simulink model "KUKAKR70"  (R2022b)
settings: Solver=ode4  StartTime=0.0  StopTime=TrajTime  FixedStep=Ts  RelTol=1e-3
values from neighbouring files (symbols this model uses):
  C = reshape([mt1,mt2,mt3,mt4,mt5,mt6,mt7,mt8,mt9,mt10,mt11,mt12,mt13,mt14,mt15,mt16,mt17],6,6)    [KR70CMatrix.m]
  X = 1200    [KR70ComputedTorque.m]
  Y = 1200    [KR70ComputedTorque.m]
  Z = 1200    [KR70ComputedTorque.m]
libraries: sm_lib x24, nesl_utility x19, simulink_extras x3
settings Model: Creator=Aboudi  LastModifiedBy=revdu
settings SolverCC: AlgebraicLoopSolver=TrustRegion
settings OptimizationCC: EnhancedBackFolding=on  PassReuseOutputArgsAs=Individual arguments  ZeroExternalMemoryAtStartup=off  ZeroInternalMemoryAtStartup=off  MaxStackSize=64  OptimizeBlockOrder=speed  DifferentSizesBufferReuse=on  OptimizationCustomize=off  EfficientTunableParamExpr=on
settings DebuggingCC: ParameterTunabilityLossMsg=error  UnconnectedInputMsg=warning  UnconnectedOutputMsg=warning  UnconnectedLineMsg=warning  SFMachineParentedDataDiag=warning
settings HardwareCC: ProdBitPerPointer=32  ProdBitPerSizeT=32  ProdBitPerPtrDiffT=32  ProdLargestAtomicFloat=None  ProdIntDivRoundTo=Undefined  ProdEndianess=Unspecified  ProdWordSize=32  ProdHWDeviceType=Generic->Unspecified (assume 32-bit Generic)
settings ModelReferenceCC: EnableRefExpFcnMdlSchedulingChecks=on
settings SFSimCC: MATLABDynamicMemAlloc=off
settings RTWCC: Description=Embedded Coder  SystemTargetFile=ert.tlc  HardwareBoard=Robot Operating System (ROS)  TLCOptions="-aInlineSetEventsForThisBaseRateFcn=TLC_FALSE -aSuppressMultiTaskScheduler=TLC_FALSE  -aRateBasedStepFcn=0"  TemplateMakefile=ert_default_tmf  Toolchain=Catkin  TargetLang=C++
settings CodeAppCC: ForceParamTrailComments=on  IgnoreCustomStorageClasses=off  OperatorAnnotations=on  SimulinkDataObjDesc=on  SFDataObjDesc=on  InsertBlockDesc=on
settings ExplorerConfigSet: InternalSimMechanicsExplorerSettings="<ExplorerConfiguration><canonicalview>aerospace</canonicalview><AnimationSetting><BasePlaybackSpeed>1.0</BasePlaybackSpeed><PlaybackSpeedFactor>1.0</PlaybackSpeedFactor></AnimationSetting><TilePanel><TileInfo><Tiles Columns=\"1\" Count=\"1\" Rows=\"1\"><Column Weight=\"1\"/><Row Weight=\"1\"/><Tile Height=\"1\" Width=\"1\" X=\"0\" Y=\"0\"/></Tiles></TileInfo><SceneInfo><SceneViewer><BGColor><R>0.60000002384185791</R><G>0.60000002384185791</G><B>0.60000002384185791</B></BGColor><Camera><DoPerspective>off</DoPerspective><Position><X>3.02357332435470916</X><Y>-3.32920549020346535</Y><Z>2.30639573599890824</Z></Position><Center><X>-0.276547744173664067</X><Y>0.35019971331948252</Y><Z>-0.00815298373152223421</Z></Center><Up><X>-0.335011191369486205</X><Y>0.267785677359949403</Y><Z>0.903359470342825488</Z></Up><ViewLimDist>1</ViewLimDist><YLim>2.19360700639605977</YLim><XLim>3.27073690415556007</XLim></Camera></SceneViewer></SceneInfo></TilePanel><MechEditorPanel><Cameras/><GfxPanelCameraMap/><VideoCreator><PlaybackSpeedRatio>1.0</PlaybackSpeedRatio><FrameRate>30</FrameRate><VideoFormat>Motion JPEG AVI</VideoFormat><FrameSize>auto</FrameSize></VideoCreator></MechEditorPanel></ExplorerConfiguration>"

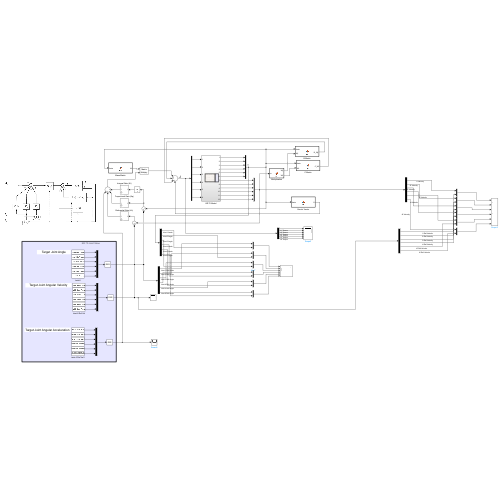
[thumbnail: Simulink's stored preview of the top-level diagram]
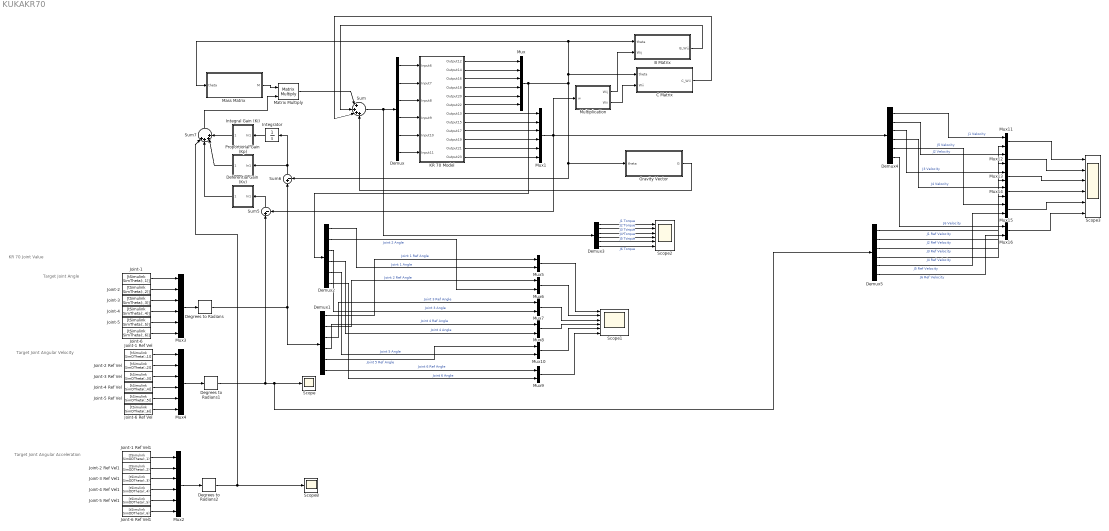
== system KUKAKR70 ==
  note: KR 70 Joint Value
  note: Target Joint Angular Velocity
  note: Target Joint Angle
  note: Target Joint Angular Acceleration
  B Matrix : MATLAB Function  TreatAsAtomicUnit=on
  C Matrix : MATLAB Function  TreatAsAtomicUnit=on
  Deferential Gain (Kv) : Subsystem  mask{Kv1=1e2, Kv2=1e2, Kv3=1e2, Kv4=1e2, Kv5=1e2, Kv6=1e3}
  Degrees to Radians : simulink_extras/Transformations/Degrees to Radians
  Degrees to Radians1 : simulink_extras/Transformations/Degrees to Radians
  Degrees to Radians2 : simulink_extras/Transformations/Degrees to Radians
  Demux{,1..5} (6 alike) : Demux  Outputs=6
  Gravity Vector : MATLAB Function  TreatAsAtomicUnit=on
  Integral Gain (Ki) : Subsystem  mask{Ki1=2e3, Ki2=2e3, Ki3=1e3, Ki4=1e2, Ki5=1e2, Ki6=1e3}
  Integrator : Integrator
  Joint-1 : FromWorkspace  VariableName=[tSimulink SimTheta(:,1)]  SampleTime=-1  OutputAfterFinalValue=Holding final value
  Joint-1 Ref Vel : FromWorkspace  VariableName=[tSimulink SimDTheta(:,1)]  SampleTime=-1  OutputAfterFinalValue=Holding final value
  Joint-1 Ref Vel1 : FromWorkspace  VariableName=[tSimulink SimDDTheta(:,1)]  SampleTime=-1  OutputAfterFinalValue=Holding final value
  Joint-2 : FromWorkspace  VariableName=[tSimulink SimTheta(:,2)]  SampleTime=-1  OutputAfterFinalValue=Holding final value
  Joint-2 Ref Vel : FromWorkspace  VariableName=[tSimulink SimDTheta(:,2)]  SampleTime=-1  OutputAfterFinalValue=Holding final value
  Joint-2 Ref Vel1 : FromWorkspace  VariableName=[tSimulink SimDDTheta(:,2)]  SampleTime=-1  OutputAfterFinalValue=Holding final value
  Joint-3 : FromWorkspace  VariableName=[tSimulink SimTheta(:,3)]  SampleTime=-1  OutputAfterFinalValue=Holding final value
  Joint-3 Ref Vel : FromWorkspace  VariableName=[tSimulink SimDTheta(:,3)]  SampleTime=-1  OutputAfterFinalValue=Holding final value
  Joint-3 Ref Vel1 : FromWorkspace  VariableName=[tSimulink SimDDTheta(:,3)]  SampleTime=-1  OutputAfterFinalValue=Holding final value
  Joint-4 : FromWorkspace  VariableName=[tSimulink SimTheta(:,4)]  SampleTime=-1  OutputAfterFinalValue=Holding final value
  Joint-4 Ref Vel : FromWorkspace  VariableName=[tSimulink SimDTheta(:,4)]  SampleTime=-1  OutputAfterFinalValue=Holding final value
  Joint-4 Ref Vel1 : FromWorkspace  VariableName=[tSimulink SimDDTheta(:,4)]  SampleTime=-1  OutputAfterFinalValue=Holding final value
  Joint-5 : FromWorkspace  VariableName=[tSimulink SimTheta(:,5)]  SampleTime=-1  OutputAfterFinalValue=Holding final value
  Joint-5 Ref Vel : FromWorkspace  VariableName=[tSimulink SimDTheta(:,5)]  SampleTime=-1  OutputAfterFinalValue=Holding final value
  Joint-5 Ref Vel1 : FromWorkspace  VariableName=[tSimulink SimDDTheta(:,5)]  SampleTime=-1  OutputAfterFinalValue=Holding final value
  Joint-6 : FromWorkspace  VariableName=[tSimulink SimTheta(:,6)]  SampleTime=-1  OutputAfterFinalValue=Holding final value
  Joint-6 Ref Vel : FromWorkspace  VariableName=[tSimulink SimDTheta(:,6)]  SampleTime=-1  OutputAfterFinalValue=Holding final value
  Joint-6 Ref Vel1 : FromWorkspace  VariableName=[tSimulink SimDDTheta(:,6)]  SampleTime=-1  OutputAfterFinalValue=Holding final value
  KR 70 Model : Subsystem
  Mass Matrix : MATLAB Function  TreatAsAtomicUnit=on
  Matrix Multiply : Product  Multiplication=Matrix(*)
  Multiplication : MATLAB Function  TreatAsAtomicUnit=on
  Mux{,1..4} (5 alike) : Mux  Inputs=6
  Mux{5..16} (12 alike) : Mux  Inputs=2
  Proportional Gain (Kp) : Subsystem  mask{K1=1e3, K2=1e3, K3=1e3, K4=3e3, K5=1e3, K6=1e6}
  Scope : Scope
  Scope1 : Scope  NumInputPorts=6
  Scope2 : Scope  NumInputPorts=6
  Scope3 : Scope  NumInputPorts=6
  Scope8 : Scope
  Sum : Sum  Inputs=|++++
  Sum5 : Sum  Inputs=|+-
  Sum6 : Sum  Inputs=|+-
  Sum7 : Sum  Inputs=|++++
  wires:
  KR 70 Model/1(Output12) -> Mux/1
  KR 70 Model/7(Output13) -> Mux1/1
  KR 70 Model/8(Output15) -> Mux1/2
  KR 70 Model/9(Output17) -> Mux1/3
  KR 70 Model/10(Output19) -> Mux1/4
  KR 70 Model/11(Output21) -> Mux1/5
  KR 70 Model/12(Output23) -> Mux1/6
  Mux1/1 -> Sum5/2, Demux4/1, Multiplication/1(w)
  Mux/1 -> Demux2/1, C Matrix/1(theta), Mass Matrix/1(theta), B Matrix/1(theta), Sum6/2, Gravity Vector/1(theta)
  Mass Matrix/1(M) -> Matrix Multiply/1
  Demux/1 -> KR 70 Model/1(Input6)
  Demux/2 -> KR 70 Model/2(Input7)
  Demux/3 -> KR 70 Model/3(Input8)
  Demux/4 -> KR 70 Model/4(Input9)
  Demux/5 -> KR 70 Model/5(Input10)
  Demux/6 -> KR 70 Model/6(Input11)
  Matrix Multiply/1 -> Sum/1
  Sum/1 -> Demux3/1, Demux/1
  Multiplication/2(Wii) -> C Matrix/2(Wii)
  Multiplication/1(Wij) -> B Matrix/2(Wij)
  Gravity Vector/1(G) -> Sum/4
  Sum6/1 -> Proportional Gain (Kp)/1(In1), Integrator/1
  Sum5/1 -> Deferential Gain (Kv)/1(In1)
  Integrator/1 -> Integral Gain (Ki)/1(In1)
  Sum7/1 -> Matrix Multiply/2
  C Matrix/1(C_Wii) -> Sum/3
  B Matrix/1(B_Wij) -> Sum/2
  Mux3/1 -> Degrees to Radians/1
  Deferential Gain (Kv)/1(Out1) -> Sum7/2
  Degrees to Radians2/1 -> Scope8/1, Sum7/1
  Mux4/1 -> Degrees to Radians1/1
  Integral Gain (Ki)/1(Out1) -> Sum7/4
  Proportional Gain (Kp)/1(Out1) -> Sum7/3
  Joint-1/1 -> Mux3/1
  Joint-2/1 -> Mux3/2
  Joint-3/1 -> Mux3/3
  Joint-4/1 -> Mux3/4
  Joint-5/1 -> Mux3/5
  Joint-6/1 -> Mux3/6
  KR 70 Model/2(Output14) -> Mux/2
  KR 70 Model/3(Output16) -> Mux/3
  KR 70 Model/4(Output18) -> Mux/4
  KR 70 Model/5(Output20) -> Mux/5
  KR 70 Model/6(Output22) -> Mux/6
  Joint-4 Ref Vel/1 -> Mux4/4
  Joint-5 Ref Vel/1 -> Mux4/5
  Joint-1 Ref Vel/1 -> Mux4/1
  Joint-6 Ref Vel/1 -> Mux4/6
  Joint-2 Ref Vel/1 -> Mux4/2
  Joint-3 Ref Vel/1 -> Mux4/3
  Degrees to Radians/1 -> Sum6/1, Demux1/1
  Degrees to Radians1/1 -> Sum5/1, Demux5/1, Scope/1
  Mux2/1 -> Degrees to Radians2/1
  Joint-2 Ref Vel1/1 -> Mux2/2
  Joint-3 Ref Vel1/1 -> Mux2/3
  Joint-6 Ref Vel1/1 -> Mux2/6
  Joint-4 Ref Vel1/1 -> Mux2/4
  Joint-1 Ref Vel1/1 -> Mux2/1
  Joint-5 Ref Vel1/1 -> Mux2/5
  Demux1/1 -> Mux5/1  "Joint 1 Ref Angle"
  Demux2/1 -> Mux5/2  "Joint 1 Angle"
  Mux5/1 -> Scope1/1
  Mux6/1 -> Scope1/2
  Mux7/1 -> Scope1/3
  Mux8/1 -> Scope1/4
  Mux10/1 -> Scope1/5
  Mux9/1 -> Scope1/6
  Demux1/2 -> Mux6/1  "Joint 2 Ref Angle"
  Demux1/3 -> Mux7/1  "Joint 3 Ref Angle"
  Demux1/4 -> Mux8/1  "Joint 4 Ref Angle"
  Demux1/5 -> Mux10/1  "Joint 5 Ref Angle"
  Demux1/6 -> Mux9/1  "Joint 6 Ref Angle"
  Demux2/2 -> Mux6/2  "Joint 2 Angle"
  Demux2/3 -> Mux7/2  "Joint 3 Angle"
  Demux2/4 -> Mux8/2  "Joint 4 Angle"
  Demux2/5 -> Mux10/2  "Joint 5 Angle"
  Demux2/6 -> Mux9/2  "Joint 6 Angle"
  Demux3/1 -> Scope2/1  "J1 Torque"
  Demux3/2 -> Scope2/2  "J2 Torque"
  Demux3/3 -> Scope2/3  "J3 Torque"
  Demux3/4 -> Scope2/4  "J4 Torque"
  Demux3/5 -> Scope2/5  "J5 Torque"
  Demux3/6 -> Scope2/6  "J6 Torque"
  Mux11/1 -> Scope3/1
  Mux12/1 -> Scope3/2
  Mux13/1 -> Scope3/3
  Mux14/1 -> Scope3/4
  Mux15/1 -> Scope3/5
  Mux16/1 -> Scope3/6
  Demux4/1 -> Mux11/1  "J1 Velocity"
  Demux4/2 -> Mux12/1  "J2 Velocity"
  Demux4/3 -> Mux13/1  "J3 Velocity"
  Demux4/4 -> Mux14/1  "J4 Velocity"
  Demux4/5 -> Mux15/1  "J5 Velocity"
  Demux4/6 -> Mux16/1  "J6 Velocity"
  Demux5/1 -> Mux11/2  "J1 Ref Velocity"
  Demux5/2 -> Mux12/2  "J2 Ref Velocity"
  Demux5/3 -> Mux13/2  "J3 Ref Velocity"
  Demux5/4 -> Mux14/2  "J4 Ref Velocity"
  Demux5/5 -> Mux15/2  "J5 Ref Velocity"
  Demux5/6 -> Mux16/2  "J6 Ref Velocity"

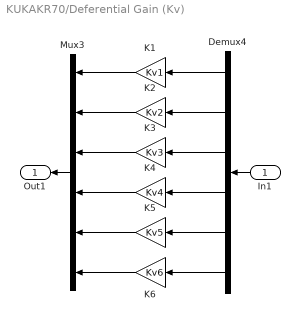
== system KUKAKR70/Deferential Gain (Kv) ==
  In1 : Inport
  Demux4 : Demux  Outputs=6
  K1 : Gain  Gain=Kv1
  K2 : Gain  Gain=Kv2
  K3 : Gain  Gain=Kv3
  K4 : Gain  Gain=Kv4
  K5 : Gain  Gain=Kv5
  K6 : Gain  Gain=Kv6
  Mux3 : Mux  Inputs=6
  Out1 : Outport
  wires:
  Demux4/3 -> K3/1
  K2/1 -> Mux3/2
  K1/1 -> Mux3/1
  K6/1 -> Mux3/6
  Demux4/2 -> K2/1
  Demux4/5 -> K5/1
  Demux4/4 -> K4/1
  Demux4/1 -> K1/1
  K4/1 -> Mux3/4
  Demux4/6 -> K6/1
  K3/1 -> Mux3/3
  K5/1 -> Mux3/5
  In1/1 -> Demux4/1
  Mux3/1 -> Out1/1

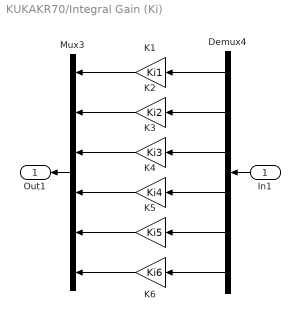
== system KUKAKR70/Integral Gain (Ki) ==
  In1 : Inport
  Demux4 : Demux  Outputs=6
  K1 : Gain  Gain=Ki1
  K2 : Gain  Gain=Ki2
  K3 : Gain  Gain=Ki3
  K4 : Gain  Gain=Ki4
  K5 : Gain  Gain=Ki5
  K6 : Gain  Gain=Ki6
  Mux3 : Mux  Inputs=6
  Out1 : Outport
  wires:
  Demux4/3 -> K3/1
  K2/1 -> Mux3/2
  K1/1 -> Mux3/1
  K6/1 -> Mux3/6
  Demux4/2 -> K2/1
  Demux4/5 -> K5/1
  Demux4/4 -> K4/1
  Demux4/1 -> K1/1
  K4/1 -> Mux3/4
  Demux4/6 -> K6/1
  K3/1 -> Mux3/3
  K5/1 -> Mux3/5
  In1/1 -> Demux4/1
  Mux3/1 -> Out1/1

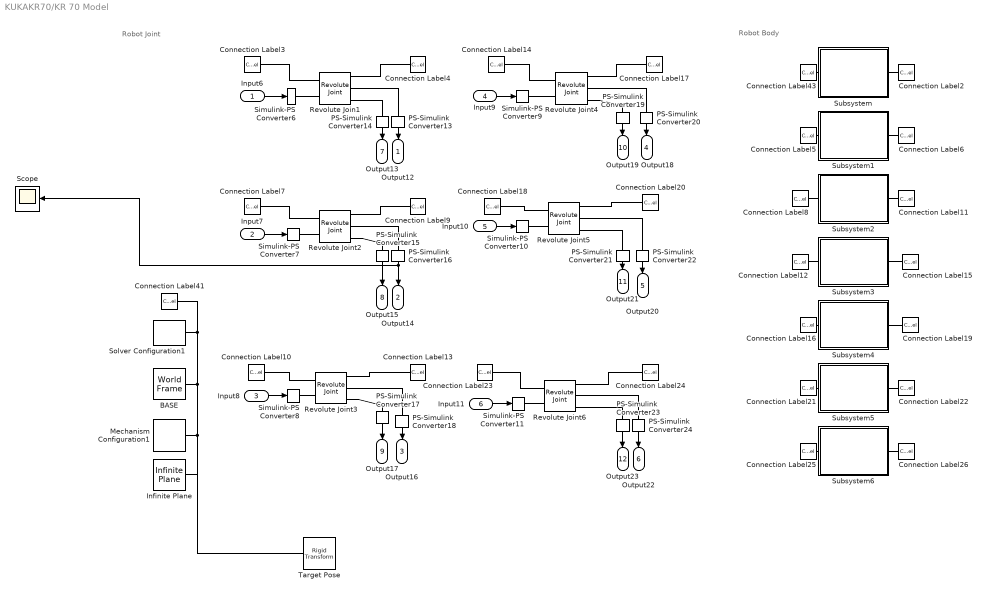
== system KUKAKR70/KR 70 Model ==
  note: Robot Joint
  note: Robot Body
  Input6 : Inport
  Input7 : Inport  Port=2
  Input8 : Inport  Port=3
  Input9 : Inport  Port=4
  Input10 : Inport  Port=5
  Input11 : Inport  Port=6
  BASE : sm_lib/Frames and Transforms/World Frame
  Connection Label10 : ConnectionLabel  Label=J3In
  Connection Label11 : ConnectionLabel  Label=J3In
  Connection Label12 : ConnectionLabel  Label=J3Out
  Connection Label13 : ConnectionLabel  Label=J3Out
  Connection Label14 : ConnectionLabel  Label=J4In
  Connection Label15 : ConnectionLabel  Label=J4In
  Connection Label16 : ConnectionLabel  Label=J4Out
  Connection Label17 : ConnectionLabel  Label=J4Out
  Connection Label18 : ConnectionLabel  Label=J5In
  Connection Label19 : ConnectionLabel  Label=J5In
  Connection Label2 : ConnectionLabel  Label=J1In
  Connection Label20 : ConnectionLabel  Label=J5Out
  Connection Label21 : ConnectionLabel  Label=J5Out
  Connection Label22 : ConnectionLabel  Label=J6In
  Connection Label23 : ConnectionLabel  Label=J6In
  Connection Label24 : ConnectionLabel  Label=J6Out
  Connection Label25 : ConnectionLabel  Label=J6Out
  Connection Label26 : ConnectionLabel  Label=EEOut
  Connection Label3 : ConnectionLabel  Label=J1In
  Connection Label4 : ConnectionLabel  Label=J1Out
  Connection Label41 : ConnectionLabel  Label=BasetoRobot
  Connection Label43 : ConnectionLabel  Label=BasetoRobot
  Connection Label5 : ConnectionLabel  Label=J1Out
  Connection Label6 : ConnectionLabel  Label=J2In
  Connection Label7 : ConnectionLabel  Label=J2In
  Connection Label8 : ConnectionLabel  Label=J2Out
  Connection Label9 : ConnectionLabel  Label=J2Out
  Infinite Plane : sm_lib/Curves and Surfaces/Infinite Plane  GraphicType=Rectangle  GraphicPlaneWidth=5  GraphicPlaneWidthUnits=m  GraphicPlaneHeight=5  GraphicPlaneHeightUnits=m  GraphicVisPropType=SimpleVisualProperties  GraphicDiffuseColor=[1 0 0]  GraphicOpacity=.25  GraphicSpecularColor=[0.5 0.5 0.5 1.0]  GraphicAmbientColor=[0.15 0.15 0.15 1.0]  GraphicEmissiveColor=[0.0 0.0 0.0 1.0]  GraphicShininess=75
  Mechanism Configuration1 : sm_lib/Utilities/Mechanism Configuration  UniformGravity=Constant  GravityVector=[0 0 -9.80665]  GravityUnits=m/s^2  LinearizationDelta=0.001  JointModeTransitionNonlinearIterations=2
  PS-Simulink Converter{13..24} (12 alike) : nesl_utility/PS-Simulink Converter  PhysicalDomain=network_engine_domain  SubClassName=ps_output  LeftPortType=input  RightPortType=output  PseudoPeriodic=off  Frequencies=[]  VectorFormat=1-D array  Unit=1  AffineConversion=off
  Revolute Join1 : sm_lib/Joints/Revolute Joint  JointMode=Normal  SenseConstraintForce=off  SenseConstraintForceX=off  SenseConstraintForceY=off  SenseConstraintForceZ=off  SenseConstraintTorque=off  SenseConstraintTorqueX=off  SenseConstraintTorqueY=off  SenseConstraintTorqueZ=off  SenseTotalForce=off  SenseTotalForceX=off  SenseTotalForceY=off  SenseTotalForceZ=off  SenseTotalTorque=off  SenseTotalTorqueX=off  SenseTotalTorqueY=off  SenseTotalTorqueZ=off  CompositeWrenchDir=FollowerOnBase  CompositeWrenchFrame=BaseFrame  EquilibriumPosition=0  EquilibriumPositionUnits=deg  SpringStiffness=0  SpringStiffnessUnits=N*m/deg  DampingCoefficient=0.5  DampingCoefficientUnits=N*m/(deg/s)  TorqueActuationMode=InputTorque  MotionActuationMode=ComputedMotion  SensePosition=on  SenseVelocity=on  SenseAcceleration=off  SenseTorqueForce=off  SenseLowerLimitTorqueForce=off  SenseUpperLimitTorqueForce=off  LowerLimitSpecify=off  LowerLimitBound=-90  LowerLimitBoundUnits=deg  LowerLimitStiffness=1e4  LowerLimitStiffnessUnits=N*m/deg  LowerLimitDamping=10  LowerLimitDampingUnits=N*m/(deg/s)  LowerLimitTransitionRegionWidth=0.1  LowerLimitTransitionRegionWidthUnits=deg  UpperLimitSpecify=off  UpperLimitBound=90  UpperLimitBoundUnits=deg  UpperLimitStiffness=1e4  UpperLimitStiffnessUnits=N*m/deg  UpperLimitDamping=10  UpperLimitDampingUnits=N*m/(deg/s)  UpperLimitTransitionRegionWidth=0.1  UpperLimitTransitionRegionWidthUnits=deg  PositionTargetSpecify=off  PositionTargetPriority=High  PositionTargetValue=0  PositionTargetValueUnits=deg  VelocityTargetSpecify=off  VelocityTargetPriority=High  VelocityTargetValue=0  VelocityTargetValueUnits=deg/s
  Revolute Joint2 : sm_lib/Joints/Revolute Joint  JointMode=Normal  SenseConstraintForce=off  SenseConstraintForceX=off  SenseConstraintForceY=off  SenseConstraintForceZ=off  SenseConstraintTorque=off  SenseConstraintTorqueX=off  SenseConstraintTorqueY=off  SenseConstraintTorqueZ=off  SenseTotalForce=off  SenseTotalForceX=off  SenseTotalForceY=off  SenseTotalForceZ=off  SenseTotalTorque=off  SenseTotalTorqueX=off  SenseTotalTorqueY=off  SenseTotalTorqueZ=off  CompositeWrenchDir=FollowerOnBase  CompositeWrenchFrame=BaseFrame  EquilibriumPosition=0  EquilibriumPositionUnits=deg  SpringStiffness=0  SpringStiffnessUnits=N*m/deg  DampingCoefficient=0.5  DampingCoefficientUnits=N*m/(deg/s)  TorqueActuationMode=InputTorque  MotionActuationMode=ComputedMotion  SensePosition=on  SenseVelocity=on  SenseAcceleration=off  SenseTorqueForce=off  SenseLowerLimitTorqueForce=off  SenseUpperLimitTorqueForce=off  LowerLimitSpecify=off  LowerLimitBound=-90  LowerLimitBoundUnits=deg  LowerLimitStiffness=1e4  LowerLimitStiffnessUnits=N*m/deg  LowerLimitDamping=10  LowerLimitDampingUnits=N*m/(deg/s)  LowerLimitTransitionRegionWidth=0.1  LowerLimitTransitionRegionWidthUnits=deg  UpperLimitSpecify=off  UpperLimitBound=90  UpperLimitBoundUnits=deg  UpperLimitStiffness=1e4  UpperLimitStiffnessUnits=N*m/deg  UpperLimitDamping=10  UpperLimitDampingUnits=N*m/(deg/s)  UpperLimitTransitionRegionWidth=0.1  UpperLimitTransitionRegionWidthUnits=deg  PositionTargetSpecify=off  PositionTargetPriority=High  PositionTargetValue=0  PositionTargetValueUnits=deg  VelocityTargetSpecify=off  VelocityTargetPriority=High  VelocityTargetValue=0  VelocityTargetValueUnits=deg/s
  Revolute Joint3 : sm_lib/Joints/Revolute Joint  JointMode=Normal  SenseConstraintForce=off  SenseConstraintForceX=off  SenseConstraintForceY=off  SenseConstraintForceZ=off  SenseConstraintTorque=off  SenseConstraintTorqueX=off  SenseConstraintTorqueY=off  SenseConstraintTorqueZ=off  SenseTotalForce=off  SenseTotalForceX=off  SenseTotalForceY=off  SenseTotalForceZ=off  SenseTotalTorque=off  SenseTotalTorqueX=off  SenseTotalTorqueY=off  SenseTotalTorqueZ=off  CompositeWrenchDir=FollowerOnBase  CompositeWrenchFrame=BaseFrame  EquilibriumPosition=0  EquilibriumPositionUnits=deg  SpringStiffness=0  SpringStiffnessUnits=N*m/deg  DampingCoefficient=0.5  DampingCoefficientUnits=N*m/(deg/s)  TorqueActuationMode=InputTorque  MotionActuationMode=ComputedMotion  SensePosition=on  SenseVelocity=on  SenseAcceleration=off  SenseTorqueForce=off  SenseLowerLimitTorqueForce=off  SenseUpperLimitTorqueForce=off  LowerLimitSpecify=off  LowerLimitBound=-90  LowerLimitBoundUnits=deg  LowerLimitStiffness=1e4  LowerLimitStiffnessUnits=N*m/deg  LowerLimitDamping=10  LowerLimitDampingUnits=N*m/(deg/s)  LowerLimitTransitionRegionWidth=0.1  LowerLimitTransitionRegionWidthUnits=deg  UpperLimitSpecify=off  UpperLimitBound=90  UpperLimitBoundUnits=deg  UpperLimitStiffness=1e4  UpperLimitStiffnessUnits=N*m/deg  UpperLimitDamping=10  UpperLimitDampingUnits=N*m/(deg/s)  UpperLimitTransitionRegionWidth=0.1  UpperLimitTransitionRegionWidthUnits=deg  PositionTargetSpecify=off  PositionTargetPriority=High  PositionTargetValue=0  PositionTargetValueUnits=deg  VelocityTargetSpecify=off  VelocityTargetPriority=High  VelocityTargetValue=0  VelocityTargetValueUnits=deg/s
  Revolute Joint4 : sm_lib/Joints/Revolute Joint  JointMode=Normal  SenseConstraintForce=off  SenseConstraintForceX=off  SenseConstraintForceY=off  SenseConstraintForceZ=off  SenseConstraintTorque=off  SenseConstraintTorqueX=off  SenseConstraintTorqueY=off  SenseConstraintTorqueZ=off  SenseTotalForce=off  SenseTotalForceX=off  SenseTotalForceY=off  SenseTotalForceZ=off  SenseTotalTorque=off  SenseTotalTorqueX=off  SenseTotalTorqueY=off  SenseTotalTorqueZ=off  CompositeWrenchDir=FollowerOnBase  CompositeWrenchFrame=BaseFrame  EquilibriumPosition=0  EquilibriumPositionUnits=deg  SpringStiffness=0  SpringStiffnessUnits=N*m/deg  DampingCoefficient=0.05  DampingCoefficientUnits=N*m/(deg/s)  TorqueActuationMode=InputTorque  MotionActuationMode=ComputedMotion  SensePosition=on  SenseVelocity=on  SenseAcceleration=off  SenseTorqueForce=off  SenseLowerLimitTorqueForce=off  SenseUpperLimitTorqueForce=off  LowerLimitSpecify=off  LowerLimitBound=-90  LowerLimitBoundUnits=deg  LowerLimitStiffness=1e4  LowerLimitStiffnessUnits=N*m/deg  LowerLimitDamping=10  LowerLimitDampingUnits=N*m/(deg/s)  LowerLimitTransitionRegionWidth=0.1  LowerLimitTransitionRegionWidthUnits=deg  UpperLimitSpecify=off  UpperLimitBound=90  UpperLimitBoundUnits=deg  UpperLimitStiffness=1e4  UpperLimitStiffnessUnits=N*m/deg  UpperLimitDamping=10  UpperLimitDampingUnits=N*m/(deg/s)  UpperLimitTransitionRegionWidth=0.1  UpperLimitTransitionRegionWidthUnits=deg  PositionTargetSpecify=off  PositionTargetPriority=High  PositionTargetValue=90  PositionTargetValueUnits=deg  VelocityTargetSpecify=off  VelocityTargetPriority=High  VelocityTargetValue=0  VelocityTargetValueUnits=deg/s
  Revolute Joint5 : sm_lib/Joints/Revolute Joint  JointMode=Normal  SenseConstraintForce=off  SenseConstraintForceX=off  SenseConstraintForceY=off  SenseConstraintForceZ=off  SenseConstraintTorque=off  SenseConstraintTorqueX=off  SenseConstraintTorqueY=off  SenseConstraintTorqueZ=off  SenseTotalForce=off  SenseTotalForceX=off  SenseTotalForceY=off  SenseTotalForceZ=off  SenseTotalTorque=off  SenseTotalTorqueX=off  SenseTotalTorqueY=off  SenseTotalTorqueZ=off  CompositeWrenchDir=FollowerOnBase  CompositeWrenchFrame=BaseFrame  EquilibriumPosition=0  EquilibriumPositionUnits=deg  SpringStiffness=0  SpringStiffnessUnits=N*m/deg  DampingCoefficient=0.05  DampingCoefficientUnits=N*m/(deg/s)  TorqueActuationMode=InputTorque  MotionActuationMode=ComputedMotion  SensePosition=on  SenseVelocity=on  SenseAcceleration=off  SenseTorqueForce=off  SenseLowerLimitTorqueForce=off  SenseUpperLimitTorqueForce=off  LowerLimitSpecify=off  LowerLimitBound=-90  LowerLimitBoundUnits=deg  LowerLimitStiffness=1e4  LowerLimitStiffnessUnits=N*m/deg  LowerLimitDamping=10  LowerLimitDampingUnits=N*m/(deg/s)  LowerLimitTransitionRegionWidth=0.1  LowerLimitTransitionRegionWidthUnits=deg  UpperLimitSpecify=off  UpperLimitBound=90  UpperLimitBoundUnits=deg  UpperLimitStiffness=1e4  UpperLimitStiffnessUnits=N*m/deg  UpperLimitDamping=10  UpperLimitDampingUnits=N*m/(deg/s)  UpperLimitTransitionRegionWidth=0.1  UpperLimitTransitionRegionWidthUnits=deg  PositionTargetSpecify=on  PositionTargetPriority=High  PositionTargetValue=90  PositionTargetValueUnits=deg  VelocityTargetSpecify=off  VelocityTargetPriority=High  VelocityTargetValue=0  VelocityTargetValueUnits=deg/s
  Revolute Joint6 : sm_lib/Joints/Revolute Joint  JointMode=Normal  SenseConstraintForce=off  SenseConstraintForceX=off  SenseConstraintForceY=off  SenseConstraintForceZ=off  SenseConstraintTorque=off  SenseConstraintTorqueX=off  SenseConstraintTorqueY=off  SenseConstraintTorqueZ=off  SenseTotalForce=off  SenseTotalForceX=off  SenseTotalForceY=off  SenseTotalForceZ=off  SenseTotalTorque=off  SenseTotalTorqueX=off  SenseTotalTorqueY=off  SenseTotalTorqueZ=off  CompositeWrenchDir=FollowerOnBase  CompositeWrenchFrame=BaseFrame  EquilibriumPosition=0  EquilibriumPositionUnits=deg  SpringStiffness=0  SpringStiffnessUnits=N*m/deg  DampingCoefficient=0.05  DampingCoefficientUnits=N*m/(deg/s)  TorqueActuationMode=InputTorque  MotionActuationMode=ComputedMotion  SensePosition=on  SenseVelocity=on  SenseAcceleration=off  SenseTorqueForce=off  SenseLowerLimitTorqueForce=off  SenseUpperLimitTorqueForce=off  LowerLimitSpecify=off  LowerLimitBound=-90  LowerLimitBoundUnits=deg  LowerLimitStiffness=1e4  LowerLimitStiffnessUnits=N*m/deg  LowerLimitDamping=10  LowerLimitDampingUnits=N*m/(deg/s)  LowerLimitTransitionRegionWidth=0.1  LowerLimitTransitionRegionWidthUnits=deg  UpperLimitSpecify=off  UpperLimitBound=90  UpperLimitBoundUnits=deg  UpperLimitStiffness=1e4  UpperLimitStiffnessUnits=N*m/deg  UpperLimitDamping=10  UpperLimitDampingUnits=N*m/(deg/s)  UpperLimitTransitionRegionWidth=0.1  UpperLimitTransitionRegionWidthUnits=deg  PositionTargetSpecify=off  PositionTargetPriority=High  PositionTargetValue=0  PositionTargetValueUnits=deg  VelocityTargetSpecify=off  VelocityTargetPriority=High  VelocityTargetValue=0  VelocityTargetValueUnits=deg/s
  Scope : Scope
  Simulink-PS Converter{6..11} (6 alike) : nesl_utility/Simulink-PS Converter  PhysicalDomain=network_engine_domain  SubClassName=ps_input  LeftPortType=input  RightPortType=output  PseudoPeriodic=off  Frequencies=[]  NoiseDistribution=none  NoiseParameters=[]  Unit=1  AffineConversion=off  FilteringAndDerivatives=provide  SimscapeFilterOrder=2  InputFilterTimeConstant=0.001  UdotUserProvided=0
  Solver Configuration1 : nesl_utility/Solver Configuration  PhysicalDomain=network_engine_domain  SubClassName=solver  LeftPortType=input  RightPortType=generic  Tones=[]  Harmonics=[]  SimulateNoise=off  Profile=off  UseLocalSampling=off  EnableSwitchedLinearOptims=on  FrequencyDomain=off  UseCCode=off  RelTol=0.001  AbsTol=1e-06  MinStep=1e-09  ToWorkspace=off  RevertToSquareIcSolve=off  NumHomotopyIterations=100  PhasorMode=off  PhasorModeNumHarmonics=1  ConsistencySolver=NEWTON_FTOL  IndexReductionMethod=DerivativeReplacement  DoDC=off  ResidualTolerance=1e-09  ConsistencyTolSource=GLOBAL  ConsistencyAbsTol=0.001  ConsistencyRelTol=0.001  ConsistencyTolFactor=0.001  UseLocalSolver=off  LocalSolverChoice=NE_BACKWARD_EULER_ADVANCER  ResolveIndetEquations=on  FunctionEvalNumThread=1  LocalSolverSampleTime=0.001  DoFixedCost=off  MaxNonlinIter=3  MaxModeIter=2  ComputeImpulses=off  ImpulseIterations=2  LinearAlgebra=Full  LinearAlgebraNumThread=0  EquationFormulation=NE_FREQUENCY_TIME_EF  DelaysMemoryBudget=1024  AutomaticFiltering=on  FilteringTimeConstant=0.001  PartitionStorageMethod=AS_NEEDED  PartitionMemoryBudget=1024  PartitionMethod=FAST
  Subsystem : Subsystem
  Subsystem1 : Subsystem
  Subsystem2 : Subsystem
  Subsystem3 : Subsystem
  Subsystem4 : Subsystem
  Subsystem5 : Subsystem
  Subsystem6 : Subsystem
  Target Pose : sm_lib/Frames and Transforms/Rigid Transform  TranslationMethod=Cartesian  TranslationStandardOffset=0  TranslationLengthUnit=mm  TranslationStandardAxis=+Z  TranslationCartesianOffset=AllTargetPose(1:3,4,end)  TranslationROffset=0  TranslationROffsetUnits=m  TranslationZOffset=0  TranslationZOffsetUnits=m  TranslationThetaOffset=0  TranslationThetaOffsetUnits=deg  RotationMethod=RotationMatrix  RotationAngleUnits=deg  RotationStandardAxis=+Z  RotationAngle=0.0  RotationArbitraryAxis=[0 0 1]  FollAlignAxisA=+X  BaseAlignAxisA=+Y  FollAlignAxisB=+Y  BaseAlignAxisB=+Z  RotationSequenceAxes=FollowerAxes  RotationSequence=XYX  RotationSequenceAngles=[0 0 0]  RotationSequenceAnglesUnits=deg  RotationMatrix=AllTargetPose(1:3,1:3,end)  Quaternion=[1 0 0 0]
  Output12 : Outport
  Output14 : Outport  Port=2
  Output16 : Outport  Port=3
  Output18 : Outport  Port=4
  Output20 : Outport  Port=5
  Output22 : Outport  Port=6
  Output13 : Outport  Port=7
  Output15 : Outport  Port=8
  Output17 : Outport  Port=9
  Output19 : Outport  Port=10
  Output21 : Outport  Port=11
  Output23 : Outport  Port=12
  wires:
  PS-Simulink Converter14/1 -> Output13/1
  Input6/1 -> Simulink-PS Converter6/1
  PS-Simulink Converter13/1 -> Output12/1
  Input7/1 -> Simulink-PS Converter7/1
  PS-Simulink Converter15/1 -> Output15/1
  PS-Simulink Converter16/1 -> Scope/1, Output14/1
  Input8/1 -> Simulink-PS Converter8/1
  PS-Simulink Converter18/1 -> Output16/1
  PS-Simulink Converter17/1 -> Output17/1
  PS-Simulink Converter20/1 -> Output18/1
  PS-Simulink Converter19/1 -> Output19/1
  Input9/1 -> Simulink-PS Converter9/1
  Input10/1 -> Simulink-PS Converter10/1
  PS-Simulink Converter21/1 -> Output21/1
  PS-Simulink Converter22/1 -> Output20/1
  PS-Simulink Converter24/1 -> Output22/1
  Input11/1 -> Simulink-PS Converter11/1
  PS-Simulink Converter23/1 -> Output23/1
  connections:
  Revolute Joint2/RConn1 -- Connection Label9/LConn1
  Revolute Join1/LConn1 -- Connection Label3/LConn1
  Revolute Joint4/RConn1 -- Connection Label17/LConn1
  Revolute Join1/RConn1 -- Connection Label4/LConn1
  Revolute Joint5/LConn1 -- Connection Label18/LConn1
  Revolute Joint6/RConn1 -- Connection Label24/LConn1
  Revolute Joint4/LConn1 -- Connection Label14/LConn1
  Revolute Joint2/LConn1 -- Connection Label7/LConn1
  Revolute Joint6/LConn1 -- Connection Label23/LConn1
  Revolute Joint5/RConn1 -- Connection Label20/LConn1
  Connection Label13/LConn1 -- Revolute Joint3/RConn1
  Revolute Join1/RConn2 -- PS-Simulink Converter13/LConn1
  Revolute Join1/RConn3 -- PS-Simulink Converter14/LConn1
  Simulink-PS Converter6/RConn1 -- Revolute Join1/LConn2
  Revolute Joint2/RConn2 -- PS-Simulink Converter16/LConn1
  Revolute Joint2/RConn3 -- PS-Simulink Converter15/LConn1
  Simulink-PS Converter7/RConn1 -- Revolute Joint2/LConn2
  Connection Label10/LConn1 -- Revolute Joint3/LConn1
  Simulink-PS Converter8/RConn1 -- Revolute Joint3/LConn2
  Revolute Joint3/RConn2 -- PS-Simulink Converter18/LConn1
  Revolute Joint3/RConn3 -- PS-Simulink Converter17/LConn1
  Revolute Joint4/RConn2 -- PS-Simulink Converter20/LConn1
  Simulink-PS Converter9/RConn1 -- Revolute Joint4/LConn2
  Revolute Joint4/RConn3 -- PS-Simulink Converter19/LConn1
  Revolute Joint5/RConn2 -- PS-Simulink Converter22/LConn1
  Revolute Joint5/RConn3 -- PS-Simulink Converter21/LConn1
  Simulink-PS Converter10/RConn1 -- Revolute Joint5/LConn2
  PS-Simulink Converter23/LConn1 -- Revolute Joint6/RConn3
  Simulink-PS Converter11/RConn1 -- Revolute Joint6/LConn2
  Revolute Joint6/RConn2 -- PS-Simulink Converter24/LConn1
  Solver Configuration1/RConn1 -- Connection Label41/LConn1 -- Target Pose/LConn1 -- Infinite Plane/LConn1 -- Mechanism Configuration1/RConn1 -- BASE/RConn1
  Connection Label6/LConn1 -- Subsystem1/RConn1
  Connection Label15/LConn1 -- Subsystem3/RConn1
  Connection Label2/LConn1 -- Subsystem/RConn1
  Connection Label25/LConn1 -- Subsystem6/LConn1
  Connection Label16/LConn1 -- Subsystem4/LConn1
  Connection Label26/LConn1 -- Subsystem6/RConn1
  Connection Label21/LConn1 -- Subsystem5/LConn1
  Connection Label22/LConn1 -- Subsystem5/RConn1
  Connection Label11/LConn1 -- Subsystem2/RConn1
  Connection Label43/LConn1 -- Subsystem/LConn1
  Connection Label19/LConn1 -- Subsystem4/RConn1
  Subsystem2/LConn1 -- Connection Label8/LConn1
  Connection Label5/LConn1 -- Subsystem1/LConn1
  Subsystem3/LConn1 -- Connection Label12/LConn1

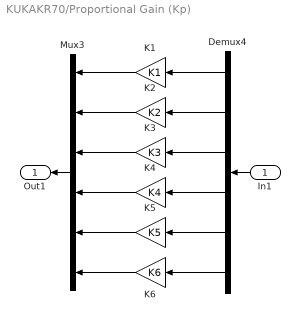
== system KUKAKR70/Proportional Gain (Kp) ==
  In1 : Inport
  Demux4 : Demux  Outputs=6
  K1 : Gain  Gain=K1
  K2 : Gain  Gain=K2
  K3 : Gain  Gain=K3
  K4 : Gain  Gain=K4
  K5 : Gain  Gain=K5
  K6 : Gain  Gain=K6
  Mux3 : Mux  Inputs=6
  Out1 : Outport
  wires:
  Demux4/3 -> K3/1
  K2/1 -> Mux3/2
  K1/1 -> Mux3/1
  K6/1 -> Mux3/6
  Demux4/2 -> K2/1
  Demux4/5 -> K5/1
  Demux4/4 -> K4/1
  Demux4/1 -> K1/1
  K4/1 -> Mux3/4
  Demux4/6 -> K6/1
  K3/1 -> Mux3/3
  K5/1 -> Mux3/5
  In1/1 -> Demux4/1
  Mux3/1 -> Out1/1

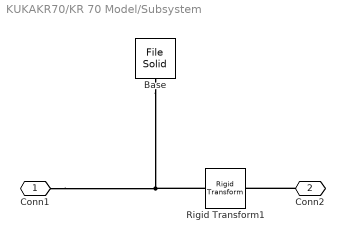
== system KUKAKR70/KR 70 Model/Subsystem ==
  Base : sm_lib/Body Elements/File Solid  ExtGeomFileName=C:\Users\revdu\OneDrive\Belgeler\GitHub\KukaKR70KinematicDynamicAnalysis\ComputedTorqueControl\stl\base.STL  UnitType=Custom  ExtGeomFileUnits=mm  StepReaderType=HEX  ExportConvexHullGeometry=off  InertiaType=Custom  Mass=92.377  MassUnits=kg  CenterOfMass=[-81.70 0.37 86.92]  CenterOfMassUnits=mm  MomentsOfInertia=[1.903 4.034 3.964]  MomentsOfInertiaUnits=kg*m^2  ProductsOfInertia=[-0.010 -0.853 0.003]  ProductsOfInertiaUnits=kg*m^2  BasedOnType=Mass  Density=3060.27  DensityUnits=kg/m^3  DoExposeReferenceFrame=on  SerializedFrames=<Frames/>  GraphicType=FromGeometry  MarkerShape=Frame  MarkerSize=10  GraphicVisPropType=SimpleVisualProperties  GraphicDiffuseColor=[0.4 0.4 0.4]  GraphicSpecularColor=[0.5 0.5 0.5 1.0]  GraphicAmbientColor=[0.15 0.15 0.15 1.0]  GraphicEmissiveColor=[0.0 0.0 0.0 1.0]  GraphicShininess=75  GraphicOpacity=1.0
  Rigid Transform1 : sm_lib/Frames and Transforms/Rigid Transform  TranslationMethod=Cartesian  TranslationStandardOffset=0  TranslationLengthUnit=mm  TranslationStandardAxis=+Z  TranslationCartesianOffset=[0 0 180]  TranslationROffset=0  TranslationROffsetUnits=m  TranslationZOffset=0  TranslationZOffsetUnits=m  TranslationThetaOffset=0  TranslationThetaOffsetUnits=deg  RotationMethod=ArbitraryAxis  RotationAngleUnits=deg  RotationStandardAxis=+Z  RotationAngle=0  RotationArbitraryAxis=[1 0 0]  FollAlignAxisA=+X  BaseAlignAxisA=+Y  FollAlignAxisB=+Y  BaseAlignAxisB=+Z  RotationSequenceAxes=FollowerAxes  RotationSequence=XYX  RotationSequenceAngles=[0 0 0]  RotationSequenceAnglesUnits=deg  RotationMatrix=[1 0 0; 0 1 0; 0 0 1]  Quaternion=[1 0 0 0]
  Conn1 : PMIOPort  Side=Left
  Conn2 : PMIOPort  Port=2  Side=Right
  connections:
  Base/RConn1 -- Rigid Transform1/LConn1 -- Conn1/RConn1
  Conn2/RConn1 -- Rigid Transform1/RConn1

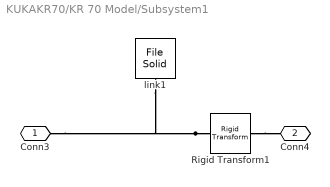
== system KUKAKR70/KR 70 Model/Subsystem1 ==
  Rigid Transform1 : sm_lib/Frames and Transforms/Rigid Transform  TranslationMethod=Cartesian  TranslationStandardOffset=0  TranslationLengthUnit=mm  TranslationStandardAxis=+Z  TranslationCartesianOffset=[175 -116.5 395]  TranslationROffset=0  TranslationROffsetUnits=m  TranslationZOffset=0  TranslationZOffsetUnits=m  TranslationThetaOffset=0  TranslationThetaOffsetUnits=deg  RotationMethod=RotationSequence  RotationAngleUnits=deg  RotationStandardAxis=+X  RotationAngle=90  RotationArbitraryAxis=[1 0 0]  FollAlignAxisA=+X  BaseAlignAxisA=+Y  FollAlignAxisB=+Y  BaseAlignAxisB=+Z  RotationSequenceAxes=FollowerAxes  RotationSequence=XYZ  RotationSequenceAngles=[90 0 0]  RotationSequenceAnglesUnits=deg  RotationMatrix=[1 0 0; 0 1 0; 0 0 1]  Quaternion=[1 0 0 0]
  link1 : sm_lib/Body Elements/File Solid  ExtGeomFileName=C:\Users\revdu\OneDrive\Belgeler\GitHub\KukaKR70KinematicDynamicAnalysis\ComputedTorqueControl\stl\link1.stl  UnitType=Custom  ExtGeomFileUnits=mm  StepReaderType=HEX  ExportConvexHullGeometry=off  InertiaType=Custom  Mass=171.666  MassUnits=kg  CenterOfMass=[60.05 11.67 237.06]  CenterOfMassUnits=mm  MomentsOfInertia=[14.911 16.857 4.672]  MomentsOfInertiaUnits=kg*m^2  ProductsOfInertia=[0.056 4.051 0.571]  ProductsOfInertiaUnits=kg*m^2  BasedOnType=DensityFromFile  Density=1000  DensityUnits=kg/m^3  DoExposeReferenceFrame=on  SerializedFrames=<Frames/>  GraphicType=FromGeometry  MarkerShape=Sphere  MarkerSize=10  GraphicVisPropType=SimpleVisualProperties  GraphicDiffuseColor=[1.0 0.6 0.2]  GraphicSpecularColor=[0.5 0.5 0.5 1.0]  GraphicAmbientColor=[0.15 0.15 0.15 1.0]  GraphicEmissiveColor=[0.0 0.0 0.0 1.0]  GraphicShininess=75  GraphicOpacity=1.0
  Conn3 : PMIOPort  Side=Left
  Conn4 : PMIOPort  Port=2  Side=Right
  connections:
  Rigid Transform1/LConn1 -- Conn3/RConn1 -- link1/RConn1
  Rigid Transform1/RConn1 -- Conn4/RConn1

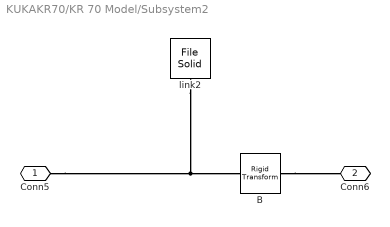
== system KUKAKR70/KR 70 Model/Subsystem2 ==
  B : sm_lib/Frames and Transforms/Rigid Transform  TranslationMethod=Cartesian  TranslationStandardOffset=0  TranslationLengthUnit=mm  TranslationStandardAxis=+Z  TranslationCartesianOffset=[890 0 63]  TranslationROffset=0  TranslationROffsetUnits=m  TranslationZOffset=0  TranslationZOffsetUnits=m  TranslationThetaOffset=0  TranslationThetaOffsetUnits=deg  RotationMethod=RotationSequence  RotationAngleUnits=deg  RotationStandardAxis=-Z  RotationAngle=90  RotationArbitraryAxis=[1 0 1]  FollAlignAxisA=+X  BaseAlignAxisA=+Y  FollAlignAxisB=+Y  BaseAlignAxisB=+Z  RotationSequenceAxes=FollowerAxes  RotationSequence=XYZ  RotationSequenceAngles=[0 0 0]  RotationSequenceAnglesUnits=deg  RotationMatrix=[1 0 0; 0 1 0; 0 0 1]  Quaternion=[1 0 0 0]
  link2 : sm_lib/Body Elements/File Solid  ExtGeomFileName=C:\Users\revdu\OneDrive\Belgeler\GitHub\KukaKR70KinematicDynamicAnalysis\ComputedTorqueControl\stl\link2.stl  UnitType=Custom  ExtGeomFileUnits=mm  StepReaderType=HEX  ExportConvexHullGeometry=off  InertiaType=Custom  Mass=61.522  MassUnits=kg  CenterOfMass=[401.52 -2.70 114.34]  CenterOfMassUnits=mm  MomentsOfInertia=[1.2 14.821 14.09]  MomentsOfInertiaUnits=kg*m^2  ProductsOfInertia=[0.009 3.165 -0.015]  ProductsOfInertiaUnits=kg*m^2  BasedOnType=DensityFromFile  Density=1000  DensityUnits=kg/m^3  DoExposeReferenceFrame=on  SerializedFrames=<Frames/>  GraphicType=FromGeometry  MarkerShape=Sphere  MarkerSize=10  GraphicVisPropType=SimpleVisualProperties  GraphicDiffuseColor=[1.0 0.6 0.2]  GraphicSpecularColor=[0.5 0.5 0.5 1.0]  GraphicAmbientColor=[0.15 0.15 0.15 1.0]  GraphicEmissiveColor=[0.0 0.0 0.0 1.0]  GraphicShininess=75  GraphicOpacity=1.0
  Conn5 : PMIOPort  Side=Left
  Conn6 : PMIOPort  Port=2  Side=Right
  connections:
  B/RConn1 -- Conn6/RConn1
  Conn5/RConn1 -- B/LConn1 -- link2/RConn1

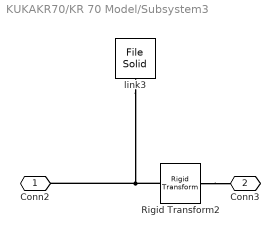
== system KUKAKR70/KR 70 Model/Subsystem3 ==
  Rigid Transform2 : sm_lib/Frames and Transforms/Rigid Transform  TranslationMethod=Cartesian  TranslationStandardOffset=0  TranslationLengthUnit=mm  TranslationStandardAxis=+Z  TranslationCartesianOffset="[50 -346.75  -179.5]"  TranslationROffset=0  TranslationROffsetUnits=m  TranslationZOffset=0  TranslationZOffsetUnits=m  TranslationThetaOffset=0  TranslationThetaOffsetUnits=deg  RotationMethod=RotationSequence  RotationAngleUnits=deg  RotationStandardAxis=+Z  RotationAngle=0.0  RotationArbitraryAxis=[0 0 1]  FollAlignAxisA=+X  BaseAlignAxisA=+Y  FollAlignAxisB=+Y  BaseAlignAxisB=+Z  RotationSequenceAxes=FollowerAxes  RotationSequence=XYZ  RotationSequenceAngles=[90 0 0]  RotationSequenceAnglesUnits=deg  RotationMatrix=[1 0 0; 0 1 0; 0 0 1]  Quaternion=[1 0 0 0]
  link3 : sm_lib/Body Elements/File Solid  ExtGeomFileName=C:\Users\revdu\OneDrive\Belgeler\GitHub\KukaKR70KinematicDynamicAnalysis\ComputedTorqueControl\stl\link3.stl  UnitType=Custom  ExtGeomFileUnits=mm  StepReaderType=HEX  ExportConvexHullGeometry=off  InertiaType=Custom  Mass=112.262  MassUnits=kg  CenterOfMass=[16.22 -30.50 -201.80]  CenterOfMassUnits=mm  MomentsOfInertia=[7.783 6.632 2.542]  MomentsOfInertiaUnits=kg*m^2  ProductsOfInertia=[-0.307 -0.0356 0.493]  ProductsOfInertiaUnits=kg*m^2  BasedOnType=DensityFromFile  Density=1000  DensityUnits=kg/m^3  DoExposeReferenceFrame=on  SerializedFrames=<Frames/>  GraphicType=FromGeometry  MarkerShape=Cube  MarkerSize=10  GraphicVisPropType=SimpleVisualProperties  GraphicDiffuseColor=[0.4 0.4 0.4]  GraphicSpecularColor=[0.5 0.5 0.5 1.0]  GraphicAmbientColor=[0.15 0.15 0.15 1.0]  GraphicEmissiveColor=[0.0 0.0 0.0 1.0]  GraphicShininess=75  GraphicOpacity=1.0
  Conn2 : PMIOPort  Side=Left
  Conn3 : PMIOPort  Port=2  Side=Right
  connections:
  Rigid Transform2/RConn1 -- Conn3/RConn1
  Rigid Transform2/LConn1 -- Conn2/RConn1 -- link3/RConn1

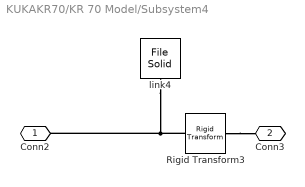
== system KUKAKR70/KR 70 Model/Subsystem4 ==
  Rigid Transform3 : sm_lib/Frames and Transforms/Rigid Transform  TranslationMethod=Cartesian  TranslationStandardOffset=0  TranslationLengthUnit=mm  TranslationStandardAxis=+Z  TranslationCartesianOffset=[0 0 688.25]  TranslationROffset=0  TranslationROffsetUnits=m  TranslationZOffset=0  TranslationZOffsetUnits=m  TranslationThetaOffset=0  TranslationThetaOffsetUnits=deg  RotationMethod=RotationSequence  RotationAngleUnits=deg  RotationStandardAxis=+Z  RotationAngle=0.0  RotationArbitraryAxis=[0 0 1]  FollAlignAxisA=+X  BaseAlignAxisA=+Y  FollAlignAxisB=+Y  BaseAlignAxisB=+Z  RotationSequenceAxes=FollowerAxes  RotationSequence=XYZ  RotationSequenceAngles=[-90 0 0]  RotationSequenceAnglesUnits=deg  RotationMatrix=[1 0 0; 0 1 0; 0 0 1]  Quaternion=[1 0 0 0]
  link4 : sm_lib/Body Elements/File Solid  ExtGeomFileName=C:\Users\revdu\OneDrive\Belgeler\GitHub\KukaKR70KinematicDynamicAnalysis\ComputedTorqueControl\stl\link4.stl  UnitType=Custom  ExtGeomFileUnits=mm  StepReaderType=HEX  ExportConvexHullGeometry=off  InertiaType=Custom  Mass=46.376  MassUnits=kg  CenterOfMass=[-0.06 -28.06 380.21]  CenterOfMassUnits=mm  MomentsOfInertia=[9.031 8.938 0.251]  MomentsOfInertiaUnits=kg*m^2  ProductsOfInertia=[0.0 -0.002 -0.798]  ProductsOfInertiaUnits=kg*m^2  BasedOnType=DensityFromFile  Density=1000  DensityUnits=kg/m^3  DoExposeReferenceFrame=on  SerializedFrames=<Frames/>  GraphicType=FromGeometry  MarkerShape=Sphere  MarkerSize=10  GraphicVisPropType=SimpleVisualProperties  GraphicDiffuseColor=[1.0 0.6 0.2]  GraphicSpecularColor=[0.5 0.5 0.5 1.0]  GraphicAmbientColor=[0.15 0.15 0.15 1.0]  GraphicEmissiveColor=[0.0 0.0 0.0 1.0]  GraphicShininess=75  GraphicOpacity=1.0
  Conn2 : PMIOPort  Side=Left
  Conn3 : PMIOPort  Port=2  Side=Right
  connections:
  Rigid Transform3/LConn1 -- link4/RConn1 -- Conn2/RConn1
  Rigid Transform3/RConn1 -- Conn3/RConn1

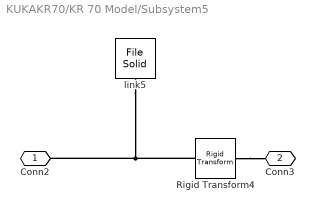
== system KUKAKR70/KR 70 Model/Subsystem5 ==
  Rigid Transform4 : sm_lib/Frames and Transforms/Rigid Transform  TranslationMethod=Cartesian  TranslationStandardOffset=0  TranslationLengthUnit=mm  TranslationStandardAxis=+Z  TranslationCartesianOffset=[0 -156.55 0]  TranslationROffset=0  TranslationROffsetUnits=m  TranslationZOffset=0  TranslationZOffsetUnits=m  TranslationThetaOffset=0  TranslationThetaOffsetUnits=deg  RotationMethod=RotationSequence  RotationAngleUnits=deg  RotationStandardAxis=+Z  RotationAngle=0.0  RotationArbitraryAxis=[0 0 1]  FollAlignAxisA=+X  BaseAlignAxisA=+Y  FollAlignAxisB=+Y  BaseAlignAxisB=+Z  RotationSequenceAxes=FollowerAxes  RotationSequence=XYZ  RotationSequenceAngles=[90 0 0]  RotationSequenceAnglesUnits=deg  RotationMatrix=[1 0 0; 0 1 0; 0 0 1]  Quaternion=[1 0 0 0]
  link5 : sm_lib/Body Elements/File Solid  ExtGeomFileName=C:\Users\revdu\OneDrive\Belgeler\GitHub\KukaKR70KinematicDynamicAnalysis\ComputedTorqueControl\stl\link5.stl  UnitType=Custom  ExtGeomFileUnits=mm  StepReaderType=HEX  ExportConvexHullGeometry=off  InertiaType=Custom  Mass=15.838  MassUnits=kg  CenterOfMass=[-0.08 -34.81 55.37]  CenterOfMassUnits=mm  MomentsOfInertia=[0.170 0.109 0.119]  MomentsOfInertiaUnits=kg*m^2  ProductsOfInertia=[0 0 -0.019]  ProductsOfInertiaUnits=kg*m^2  BasedOnType=DensityFromFile  Density=1000  DensityUnits=kg/m^3  DoExposeReferenceFrame=on  SerializedFrames=<Frames/>  GraphicType=FromGeometry  MarkerShape=Sphere  MarkerSize=10  GraphicVisPropType=SimpleVisualProperties  GraphicDiffuseColor=[0.4 0.4 0.4]  GraphicSpecularColor=[0.5 0.5 0.5 1.0]  GraphicAmbientColor=[0.15 0.15 0.15 1.0]  GraphicEmissiveColor=[0.0 0.0 0.0 1.0]  GraphicShininess=75  GraphicOpacity=1.0
  Conn2 : PMIOPort  Side=Left
  Conn3 : PMIOPort  Port=2  Side=Right
  connections:
  Rigid Transform4/LConn1 -- Conn2/RConn1 -- link5/RConn1
  Rigid Transform4/RConn1 -- Conn3/RConn1

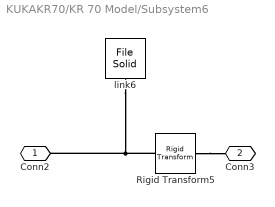
== system KUKAKR70/KR 70 Model/Subsystem6 ==
  Rigid Transform5 : sm_lib/Frames and Transforms/Rigid Transform  TranslationMethod=Cartesian  TranslationStandardOffset=0  TranslationLengthUnit=mm  TranslationStandardAxis=+Z  TranslationCartesianOffset=[0 0 30]  TranslationROffset=0  TranslationROffsetUnits=m  TranslationZOffset=0  TranslationZOffsetUnits=m  TranslationThetaOffset=0  TranslationThetaOffsetUnits=deg  RotationMethod=RotationSequence  RotationAngleUnits=deg  RotationStandardAxis=+Z  RotationAngle=0.0  RotationArbitraryAxis=[0 0 1]  FollAlignAxisA=+X  BaseAlignAxisA=+Y  FollAlignAxisB=+Y  BaseAlignAxisB=+Z  RotationSequenceAxes=FollowerAxes  RotationSequence=XYZ  RotationSequenceAngles=[0 0 0]  RotationSequenceAnglesUnits=deg  RotationMatrix=[1 0 0; 0 1 0; 0 0 1]  Quaternion=[1 0 0 0]
  link6 : sm_lib/Body Elements/File Solid  ExtGeomFileName=C:\Users\revdu\OneDrive\Belgeler\GitHub\KukaKR70KinematicDynamicAnalysis\ComputedTorqueControl\stl\link6.stl  UnitType=Custom  ExtGeomFileUnits=mm  StepReaderType=HEX  ExportConvexHullGeometry=off  InertiaType=Custom  Mass=1.111  MassUnits=kg  CenterOfMass=[-0.04 0 11.43]  CenterOfMassUnits=mm  MomentsOfInertia=[0.001 0.001 0.002]  MomentsOfInertiaUnits=kg*m^2  ProductsOfInertia=[0 0 0]  ProductsOfInertiaUnits=kg*m^2  BasedOnType=DensityFromFile  Density=1000  DensityUnits=kg/m^3  DoExposeReferenceFrame=on  SerializedFrames=<Frames/>  GraphicType=FromGeometry  MarkerShape=Sphere  MarkerSize=10  GraphicVisPropType=SimpleVisualProperties  GraphicDiffuseColor=[1.0 0.6 0.0]  GraphicSpecularColor=[0.5 0.5 0.5 1.0]  GraphicAmbientColor=[0.15 0.15 0.15 1.0]  GraphicEmissiveColor=[0.0 0.0 0.0 1.0]  GraphicShininess=75  GraphicOpacity=1.0
  Conn2 : PMIOPort  Side=Left
  Conn3 : PMIOPort  Port=2  Side=Right
  connections:
  Rigid Transform5/RConn1 -- Conn3/RConn1
  Rigid Transform5/LConn1 -- Conn2/RConn1 -- link6/RConn1

== matlab function KUKAKR70/C Matrix ==
  data: C_Wii output; theta input; Wii input
function C_Wii = fcn (theta, Wii)
theta1 =  theta(1);
theta2 =  theta(2);
theta3 =  theta(3);
theta4 =  theta(4);
theta5 =  theta(5);
theta6 =  theta(6);

C = KR70CMatrix(theta1,theta2,theta3,theta4,theta5,theta6);

C_Wii = C*Wii;

== matlab function KUKAKR70/Multiplication ==
  data: Wij output; Wii output; w input
function [Wij, Wii] = fcn(w)

Wij = [w(1)*w(2);
        w(1)*w(3);
        w(1)*w(4);
        w(1)*w(5);
        w(1)*w(6);
        w(2)*w(3);
        w(2)*w(4);
        w(2)*w(5);
        w(2)*w(6);
        w(3)*w(4);
        w(3)*w(5);
        w(3)*w(6);
        w(4)*w(5);
        w(4)*w(6);
        w(5)*w(6);];
    
Wii = [w(1)*w(1);
       w(2)*w(2);
       w(3)*w(3);
       w(4)*w(4);
       w(5)*w(5);
       w(6)*w(6);];
    
end

== matlab function KUKAKR70/B Matrix ==
  data: B_Wij output; theta input; Wij input
function B_Wij = fcn (theta, Wij)
theta1 =  theta(1);
theta2 =  theta(2);
theta3 =  theta(3);
theta4 =  theta(4);
theta5 =  theta(5);
theta6 =  theta(6);


B = KR70BMatrix(theta1,theta2,theta3,theta4,theta5,theta6);

B_Wij = B*Wij;

== matlab function KUKAKR70/Mass Matrix ==
  data: M output; theta input
function M = fcn (theta)
theta1 =  theta(1);
theta2 =  theta(2);
theta3 =  theta(3);
theta4 =  theta(4);
theta5 =  theta(5);
theta6 =  theta(6);

M = KR70MassMatrix(theta1, theta2, theta3, theta4, theta5, theta6);

== matlab function KUKAKR70/Gravity Vector ==
  data: G output; theta input
function G = fcn (theta)
theta1 =  theta(1);
theta2 =  theta(2);
theta3 =  theta(3);
theta4 =  theta(4);
theta5 =  theta(5);
theta6 =  theta(6);

G = KR70GravityVector(theta2,theta3,theta4,theta5,theta6);
